simulink model "Demuxexp1"  (R2015b)
settings: Solver=VariableStepAuto  StartTime=0.0  StopTime=10.0  RelTol=1e-3
settings Model: Creator=LUBO  LastModifiedBy=LUBO

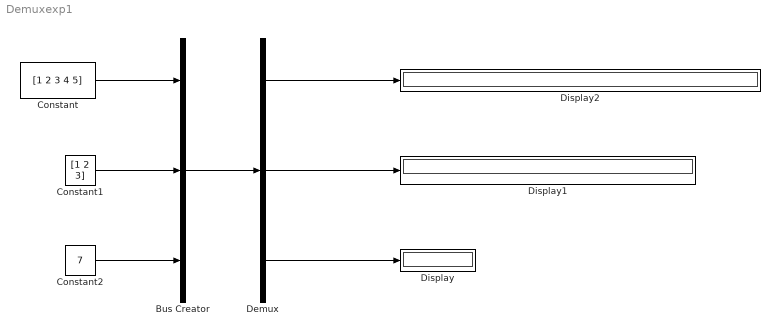
== system Demuxexp1 ==
  Bus Creator : BusCreator  Inputs=3
  Constant : Constant  Value=[1 2 3 4 5]
  Constant1 : Constant  Value=[1 2 3]
  Constant2 : Constant  Value=7
  Demux : Demux  Outputs=3  BusSelectionMode=on
  Display : Display
  Display1 : Display
  Display2 : Display
  wires:
  Demux/2 -> Display1/1
  Demux/1 -> Display2/1
  Constant/1 -> Bus Creator/1
  Constant1/1 -> Bus Creator/2
  Constant2/1 -> Bus Creator/3
  Bus Creator/1 -> Demux/1
  Demux/3 -> Display/1
